simulink model "bh_2dof_ODE_model"  (R2017a)
settings: Solver=ode45  StartTime=0.0  StopTime=20  RelTol=1e-5  EnableMultiTasking=on
PreLoadFcn:
  | bh_script_2dof_params
values from neighbouring files (symbols this model uses):
  c1 = 20    [bh_2dof_MATLAB_analysis.m]
  c2 = 50    [bh_2dof_MATLAB_analysis.m]
  c3 = 10    [bh_2dof_MATLAB_analysis.m]
  k1 = 1000    [bh_2dof_MATLAB_analysis.m]
  k2 = 500    [bh_2dof_MATLAB_analysis.m]
  k3 = 100    [bh_2dof_MATLAB_analysis.m]
  m1 = 10    [bh_2dof_MATLAB_analysis.m]
  m2 = 1    [bh_2dof_MATLAB_analysis.m]
undefined symbols (not defined in the file or in its folder): Cm_mat, init_pos_col, init_vel_col, init_x1, init_x1dot, init_x2, init_x2dot, Km_mat, Mm_mat
settings Model: Creator=bhorton  LastModifiedBy=bhorton
settings OptimizationCC: LifeSpan=inf
settings DebuggingCC: SFUnexpectedBacktrackingDiag=warning  SFNoUnconditionalDefaultTransitionDiag=warning  SFExecutionAtInitializationDiag=none
settings GRTTargetCC: TargetLangStandard=C89/C90 (ANSI)  GeneratePreprocessorConditionals=Disable all
settings ConfigComp: CovMetricSettings=dw  CovHtmlReporting=on  CovSaveCumulativeToWorkspaceVar=on  CovSaveSingleToWorkspaceVar=on  CovExternalEMLEnable=off

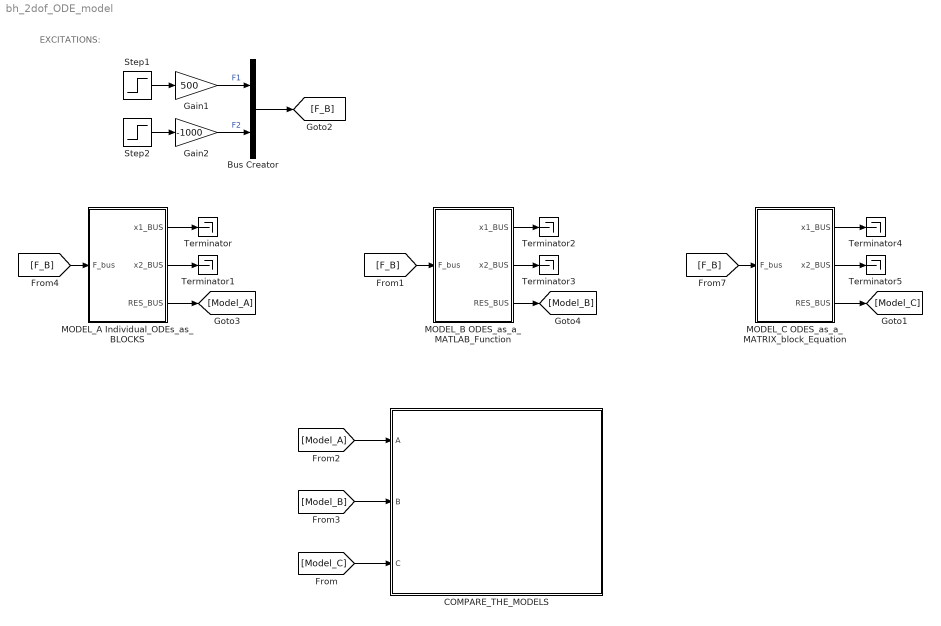
== system bh_2dof_ODE_model ==
  note: EXCITATIONS:
  Bus Creator : BusCreator  Inputs=2
  COMPARE_THE_MODELS : Subsystem
  Gain1 : Gain  Gain=500
  Gain2 : Gain  Gain=-1000
  MODEL_A Individual_ODEs_as_BLOCKS : Subsystem
  "MODEL_B ODES_as_a_MATLAB_Function " : Subsystem
  MODEL_C ODES_as_a_MATRIX_block_Equation : Subsystem
  Step1 : Step  Time=5  SampleTime=0
      settings: AttributesFormatString=Step @ T=%<Time>
  Step2 : Step  Time=10  SampleTime=0
      settings: AttributesFormatString=Step @ T=%<Time>
  Terminator{,1..5} (6 alike) : Terminator
  wires:
  Step1/1 -> Gain1/1
  Gain1/1 -> Bus Creator/1  "F1"
  Step2/1 -> Gain2/1
  Gain2/1 -> Bus Creator/2  "F2"
  Bus Creator/1 -> [F_B]
  [F_B] -> MODEL_A Individual_ODEs_as_BLOCKS/1(F_bus)
  [F_B] -> "MODEL_B ODES_as_a_MATLAB_Function "/1(F_bus)
  [F_B] -> MODEL_C ODES_as_a_MATRIX_block_Equation/1(F_bus)
  MODEL_A Individual_ODEs_as_BLOCKS/3(RES_BUS) -> [Model_A]
  "MODEL_B ODES_as_a_MATLAB_Function "/3(RES_BUS) -> [Model_B]
  MODEL_C ODES_as_a_MATRIX_block_Equation/3(RES_BUS) -> [Model_C]
  [Model_A] -> COMPARE_THE_MODELS/1(A)
  [Model_B] -> COMPARE_THE_MODELS/2(B)
  [Model_C] -> COMPARE_THE_MODELS/3(C)
  MODEL_A Individual_ODEs_as_BLOCKS/1(x1_BUS) -> Terminator/1
  MODEL_A Individual_ODEs_as_BLOCKS/2(x2_BUS) -> Terminator1/1
  "MODEL_B ODES_as_a_MATLAB_Function "/1(x1_BUS) -> Terminator2/1
  "MODEL_B ODES_as_a_MATLAB_Function "/2(x2_BUS) -> Terminator3/1
  MODEL_C ODES_as_a_MATRIX_block_Equation/2(x2_BUS) -> Terminator5/1
  MODEL_C ODES_as_a_MATRIX_block_Equation/1(x1_BUS) -> Terminator4/1

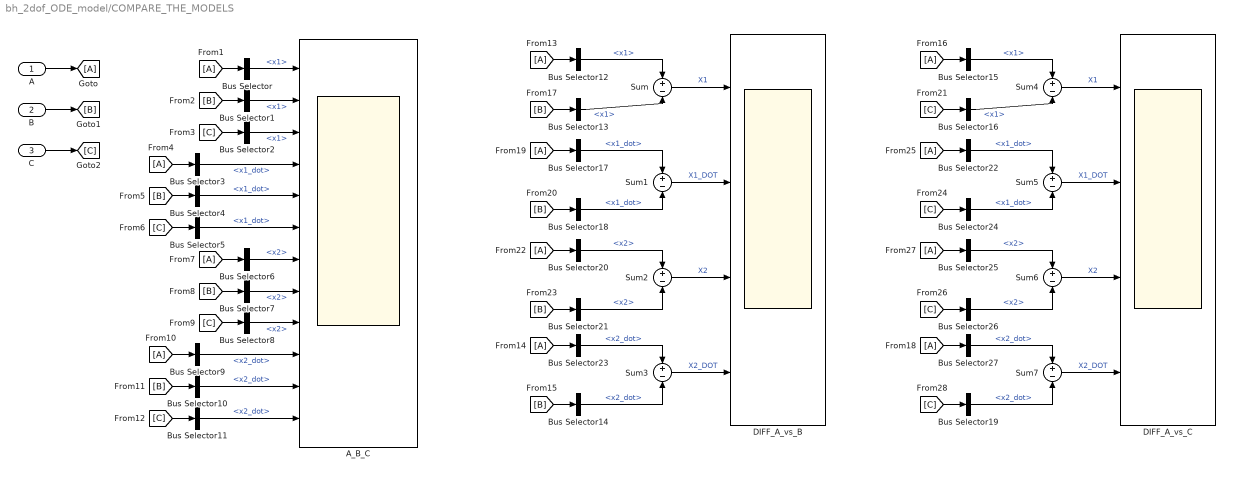
== system bh_2dof_ODE_model/COMPARE_THE_MODELS ==
  A : Inport
  B : Inport  Port=2
  C : Inport  Port=3
  A_B_C : Scope  NumInputPorts=12
  Bus Selector{,1..2,12..13,15..16} (7 alike) : BusSelector  OutputSignals=x1_BUS.x1
  Bus Selector{9..11,14,19,23,27} (7 alike) : BusSelector  OutputSignals=x2_BUS.x2_dot
  Bus Selector{3..5,17..18,22,24} (7 alike) : BusSelector  OutputSignals=x1_BUS.x1_dot
  Bus Selector{6..8,20..21,25..26} (7 alike) : BusSelector  OutputSignals=x2_BUS.x2
  DIFF_A_vs_B : Scope  NumInputPorts=4
  DIFF_A_vs_C : Scope  NumInputPorts=4
  Sum{,1..7} (8 alike) : Sum  Inputs=+|-
  wires:
  A/1 -> [A]
  B/1 -> [B]
  C/1 -> [C]
  [A] -> Bus Selector/1
  [B] -> Bus Selector1/1
  [C] -> Bus Selector2/1
  Bus Selector2/1 -> A_B_C/3  "<x1>"
  Bus Selector1/1 -> A_B_C/2  "<x1>"
  Bus Selector/1 -> A_B_C/1  "<x1>"
  Bus Selector3/1 -> A_B_C/4  "<x1_dot>"
  [A] -> Bus Selector3/1
  [C] -> Bus Selector5/1
  [B] -> Bus Selector4/1
  Bus Selector4/1 -> A_B_C/5  "<x1_dot>"
  Bus Selector5/1 -> A_B_C/6  "<x1_dot>"
  [B] -> Bus Selector7/1
  Bus Selector6/1 -> A_B_C/7  "<x2>"
  [C] -> Bus Selector8/1
  [A] -> Bus Selector6/1
  Bus Selector7/1 -> A_B_C/8  "<x2>"
  Bus Selector8/1 -> A_B_C/9  "<x2>"
  Bus Selector9/1 -> A_B_C/10  "<x2_dot>"
  [A] -> Bus Selector9/1
  [C] -> Bus Selector11/1
  [B] -> Bus Selector10/1
  Bus Selector10/1 -> A_B_C/11  "<x2_dot>"
  Bus Selector11/1 -> A_B_C/12  "<x2_dot>"
  Sum3/1 -> DIFF_A_vs_B/4  "X2_DOT"
  Bus Selector12/1 -> Sum/1  "<x1>"
  [A] -> Bus Selector20/1
  [A] -> Bus Selector17/1
  Bus Selector13/1 -> Sum/2  "<x1>"
  [B] -> Bus Selector14/1
  Bus Selector20/1 -> Sum2/1  "<x2>"
  [A] -> Bus Selector23/1
  [B] -> Bus Selector18/1
  [B] -> Bus Selector13/1
  [B] -> Bus Selector21/1
  Bus Selector14/1 -> Sum3/2  "<x2_dot>"
  Bus Selector18/1 -> Sum1/2  "<x1_dot>"
  Sum2/1 -> DIFF_A_vs_B/3  "X2"
  Bus Selector23/1 -> Sum3/1  "<x2_dot>"
  Sum/1 -> DIFF_A_vs_B/1  "X1"
  Sum1/1 -> DIFF_A_vs_B/2  "X1_DOT"
  Bus Selector17/1 -> Sum1/1  "<x1_dot>"
  Bus Selector21/1 -> Sum2/2  "<x2>"
  [A] -> Bus Selector12/1
  Bus Selector26/1 -> Sum6/2  "<x2>"
  Bus Selector15/1 -> Sum4/1  "<x1>"
  [A] -> Bus Selector15/1
  [C] -> Bus Selector19/1
  [C] -> Bus Selector26/1
  [C] -> Bus Selector16/1
  Sum4/1 -> DIFF_A_vs_C/1  "X1"
  Bus Selector19/1 -> Sum7/2  "<x2_dot>"
  [A] -> Bus Selector22/1
  Sum6/1 -> DIFF_A_vs_C/3  "X2"
  Bus Selector16/1 -> Sum4/2  "<x1>"
  Bus Selector25/1 -> Sum6/1  "<x2>"
  [A] -> Bus Selector27/1
  Bus Selector24/1 -> Sum5/2  "<x1_dot>"
  [A] -> Bus Selector25/1
  [C] -> Bus Selector24/1
  Bus Selector27/1 -> Sum7/1  "<x2_dot>"
  Bus Selector22/1 -> Sum5/1  "<x1_dot>"
  Sum5/1 -> DIFF_A_vs_C/2  "X1_DOT"
  Sum7/1 -> DIFF_A_vs_C/4  "X2_DOT"

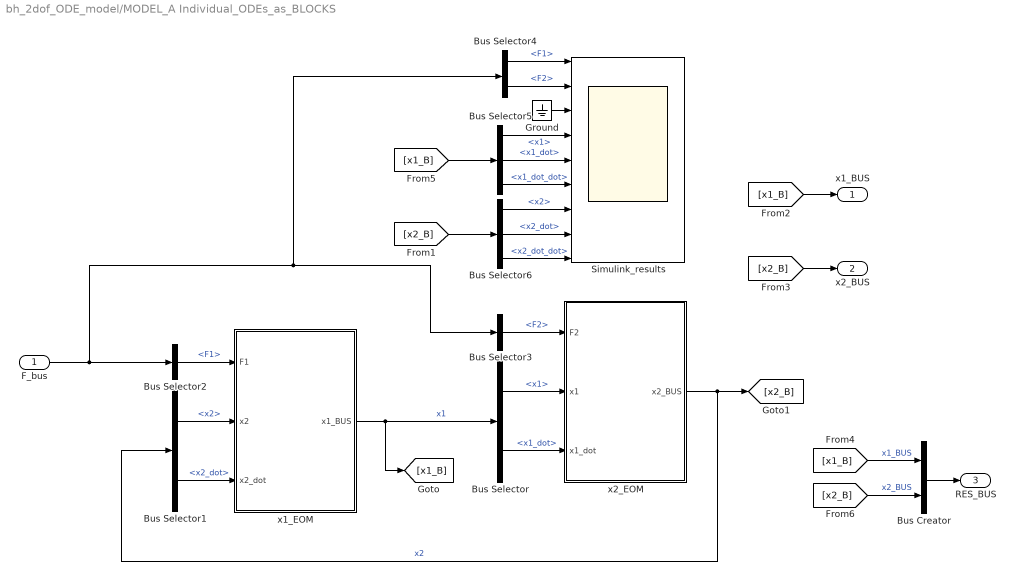
== system bh_2dof_ODE_model/MODEL_A Individual_ODEs_as_BLOCKS ==
  F_bus : Inport
  Bus Creator : BusCreator  Inputs=2
  Bus Selector : BusSelector  OutputSignals=x1,x1_dot
  Bus Selector1 : BusSelector  OutputSignals=x2,x2_dot
  Bus Selector2 : BusSelector  OutputSignals=F1
  Bus Selector3 : BusSelector  OutputSignals=F2
  Bus Selector4 : BusSelector  OutputSignals=F1,F2
  Bus Selector5 : BusSelector  OutputSignals=x1,x1_dot,x1_dot_dot
  Bus Selector6 : BusSelector  OutputSignals=x2,x2_dot,x2_dot_dot
  Ground : Ground
  Simulink_results : Scope  NumInputPorts=9
  x1_EOM : Subsystem
  x2_EOM : Subsystem
  x1_BUS : Outport
  x2_BUS : Outport  Port=2
  RES_BUS : Outport  Port=3
  wires:
  Bus Selector/2 -> x2_EOM/3(x1_dot)  "<x1_dot>"
  Bus Selector/1 -> x2_EOM/2(x1)  "<x1>"
  Bus Selector1/1 -> x1_EOM/2(x2)  "<x2>"
  Bus Selector1/2 -> x1_EOM/3(x2_dot)  "<x2_dot>"
  x1_EOM/1(x1_BUS) -> [x1_B], Bus Selector/1  "x1"
  x2_EOM/1(x2_BUS) -> Bus Selector1/1, [x2_B]  "x2"
  Bus Selector2/1 -> x1_EOM/1(F1)  "<F1>"
  Bus Selector3/1 -> x2_EOM/1(F2)  "<F2>"
  F_bus/1 -> Bus Selector4/1, Bus Selector3/1, Bus Selector2/1
  Bus Selector4/1 -> Simulink_results/1  "<F1>"
  Bus Selector4/2 -> Simulink_results/2  "<F2>"
  Ground/1 -> Simulink_results/3
  [x1_B] -> Bus Selector5/1
  Bus Selector5/3 -> Simulink_results/6  "<x1_dot_dot>"
  Bus Selector5/2 -> Simulink_results/5  "<x1_dot>"
  Bus Selector5/1 -> Simulink_results/4  "<x1>"
  Bus Selector6/1 -> Simulink_results/7  "<x2>"
  Bus Selector6/2 -> Simulink_results/8  "<x2_dot>"
  Bus Selector6/3 -> Simulink_results/9  "<x2_dot_dot>"
  [x2_B] -> Bus Selector6/1
  [x1_B] -> x1_BUS/1
  [x2_B] -> x2_BUS/1
  Bus Creator/1 -> RES_BUS/1
  [x1_B] -> Bus Creator/1  "x1_BUS"
  [x2_B] -> Bus Creator/2  "x2_BUS"

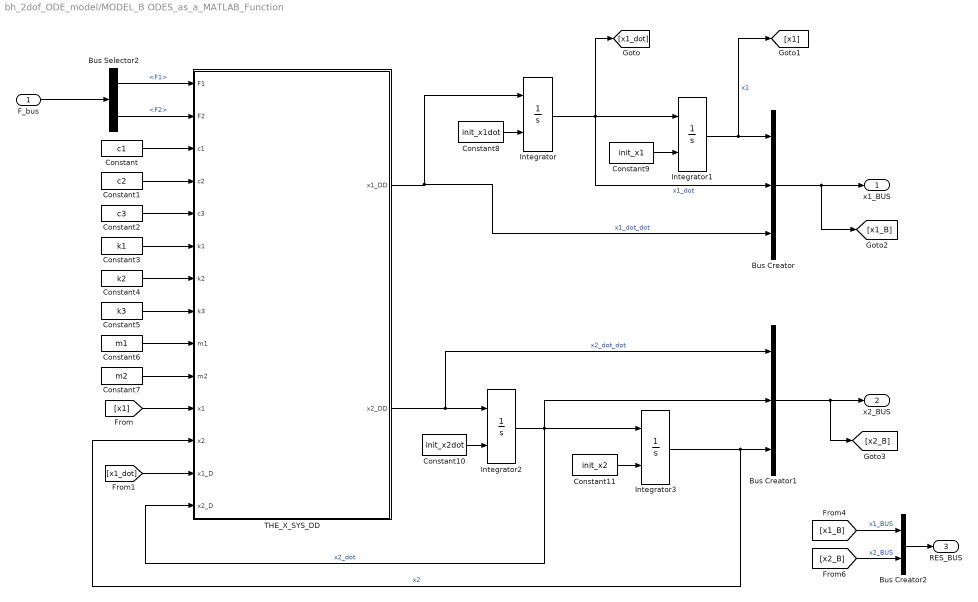
== system bh_2dof_ODE_model/MODEL_B ODES_as_a_MATLAB_Function  ==
  F_bus : Inport
  Bus Creator : BusCreator  Inputs=3
  Bus Creator1 : BusCreator  Inputs=3
  Bus Creator2 : BusCreator  Inputs=2
  Bus Selector2 : BusSelector  OutputSignals=F1,F2
  Constant : Constant  Value=c1
  Constant1 : Constant  Value=c2
  Constant10 : Constant  Value=init_x2dot
  Constant11 : Constant  Value=init_x2
  Constant2 : Constant  Value=c3
  Constant3 : Constant  Value=k1
  Constant4 : Constant  Value=k2
  Constant5 : Constant  Value=k3
  Constant6 : Constant  Value=m1
  Constant7 : Constant  Value=m2
  Constant8 : Constant  Value=init_x1dot
  Constant9 : Constant  Value=init_x1
  Integrator{,1..3} (4 alike) : Integrator  InitialConditionSource=external
  THE_X_SYS_DD : MATLAB Function  TreatAsAtomicUnit=on
  x1_BUS : Outport
  x2_BUS : Outport  Port=2
  RES_BUS : Outport  Port=3
  wires:
  F_bus/1 -> Bus Selector2/1
  Bus Selector2/2 -> THE_X_SYS_DD/2(F2)  "<F2>"
  Bus Selector2/1 -> THE_X_SYS_DD/1(F1)  "<F1>"
  Constant7/1 -> THE_X_SYS_DD/10(m2)
  Constant6/1 -> THE_X_SYS_DD/9(m1)
  Constant5/1 -> THE_X_SYS_DD/8(k3)
  Constant4/1 -> THE_X_SYS_DD/7(k2)
  Constant3/1 -> THE_X_SYS_DD/6(k1)
  Constant2/1 -> THE_X_SYS_DD/5(c3)
  Constant1/1 -> THE_X_SYS_DD/4(c2)
  Constant/1 -> THE_X_SYS_DD/3(c1)
  Bus Creator/1 -> [x1_B], x1_BUS/1
  THE_X_SYS_DD/1(x1_DD) -> Bus Creator/3, Integrator/1  "x1_dot_dot"
  Constant9/1 -> Integrator1/2
  Constant8/1 -> Integrator/2
  Integrator/1 -> [x1_dot], Bus Creator/2, Integrator1/1  "x1_dot"
  Constant11/1 -> Integrator3/2
  THE_X_SYS_DD/2(x2_DD) -> Bus Creator1/1, Integrator2/1  "x2_dot_dot"
  Bus Creator1/1 -> [x2_B], x2_BUS/1
  Integrator3/1 -> Bus Creator1/3, THE_X_SYS_DD/12(x2)  "x2"
  Constant10/1 -> Integrator2/2
  Integrator2/1 -> Bus Creator1/2, Integrator3/1, THE_X_SYS_DD/14(x2_D)  "x2_dot"
  Integrator1/1 -> [x1], Bus Creator/1  "x1"
  [x1] -> THE_X_SYS_DD/11(x1)
  [x1_dot] -> THE_X_SYS_DD/13(x1_D)
  [x1_B] -> Bus Creator2/1  "x1_BUS"
  [x2_B] -> Bus Creator2/2  "x2_BUS"
  Bus Creator2/1 -> RES_BUS/1

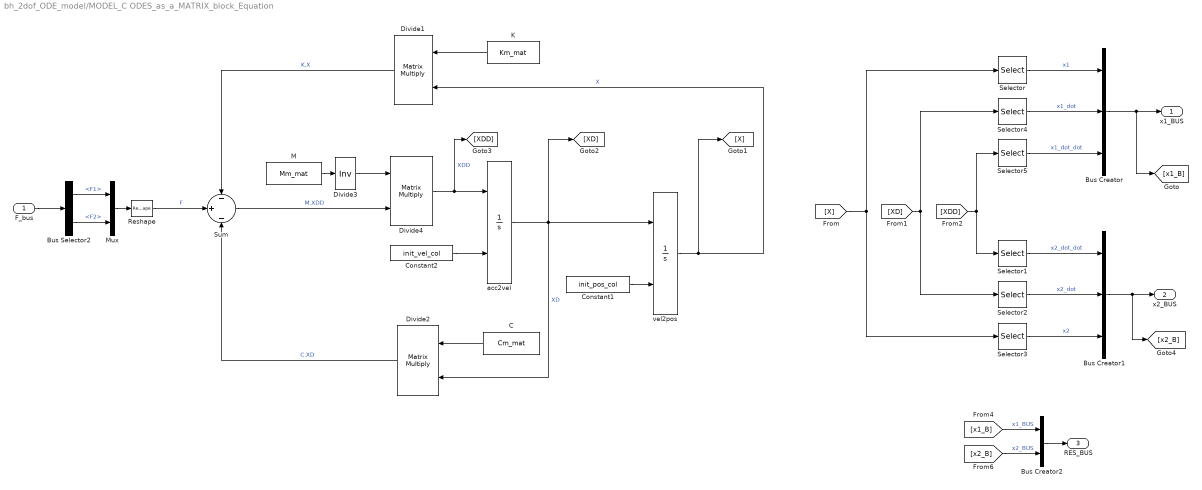
== system bh_2dof_ODE_model/MODEL_C ODES_as_a_MATRIX_block_Equation ==
  F_bus : Inport
  Bus Creator : BusCreator  Inputs=3
  Bus Creator1 : BusCreator  Inputs=3
  Bus Creator2 : BusCreator  Inputs=2
  Bus Selector2 : BusSelector  OutputSignals=F1,F2
  C : Constant  Value=Cm_mat
  Constant1 : Constant  Value=init_pos_col
  Constant2 : Constant  Value=init_vel_col
  Divide1 : Product  Multiplication=Matrix(*)
  Divide2 : Product  Multiplication=Matrix(*)
  Divide3 : Product  Inputs=/  Multiplication=Matrix(*)
  Divide4 : Product  Multiplication=Matrix(*)
  K : Constant  Value=Km_mat
  M : Constant  Value=Mm_mat
  Mux : Mux  Inputs=2
  Reshape : Reshape  OutputDimensionality=Column vector (2-D)
  Selector : Selector  InputPortWidth=2  IndexOptions=Index vector (dialog)  Indices=[1 ]  OutputSizes=1
  Selector1 : Selector  InputPortWidth=2  IndexOptions=Index vector (dialog)  Indices=[2]  OutputSizes=1
  Selector2 : Selector  InputPortWidth=2  IndexOptions=Index vector (dialog)  Indices=[2]  OutputSizes=1
  Selector3 : Selector  InputPortWidth=2  IndexOptions=Index vector (dialog)  Indices=[2]  OutputSizes=1
  Selector4 : Selector  InputPortWidth=2  IndexOptions=Index vector (dialog)  Indices=[1 ]  OutputSizes=1
  Selector5 : Selector  InputPortWidth=2  IndexOptions=Index vector (dialog)  Indices=[1 ]  OutputSizes=1
  Sum : Sum  Inputs=-|+|-
  acc2vel : Integrator  InitialConditionSource=external
  vel2pos : Integrator  InitialConditionSource=external
  x1_BUS : Outport
  x2_BUS : Outport  Port=2
  RES_BUS : Outport  Port=3
  wires:
  F_bus/1 -> Bus Selector2/1
  Bus Selector2/2 -> Mux/2  "<F2>"
  Bus Selector2/1 -> Mux/1  "<F1>"
  Bus Creator/1 -> [x1_B], x1_BUS/1
  Bus Creator1/1 -> [x2_B], x2_BUS/1
  Mux/1 -> Reshape/1
  Reshape/1 -> Sum/2  "F"
  K/1 -> Divide1/1
  C/1 -> Divide2/1
  Divide2/1 -> Sum/3  "C.XD"
  Divide1/1 -> Sum/1  "K.X"
  Sum/1 -> Divide4/2  "M.XDD"
  M/1 -> Divide3/1
  Divide3/1 -> Divide4/1
  Divide4/1 -> [XDD], acc2vel/1  "XDD"
  Constant2/1 -> acc2vel/2
  acc2vel/1 -> [XD], vel2pos/1, Divide2/2  "XD"
  Constant1/1 -> vel2pos/2
  vel2pos/1 -> [X], Divide1/2  "X"
  Selector5/1 -> Bus Creator/3  "x1_dot_dot"
  Selector4/1 -> Bus Creator/2  "x1_dot"
  Selector/1 -> Bus Creator/1  "x1"
  [XDD] -> Selector5/1, Selector1/1
  [XD] -> Selector2/1, Selector4/1
  [X] -> Selector/1, Selector3/1
  Selector1/1 -> Bus Creator1/1  "x2_dot_dot"
  Selector2/1 -> Bus Creator1/2  "x2_dot"
  Selector3/1 -> Bus Creator1/3  "x2"
  Bus Creator2/1 -> RES_BUS/1
  [x1_B] -> Bus Creator2/1  "x1_BUS"
  [x2_B] -> Bus Creator2/2  "x2_BUS"

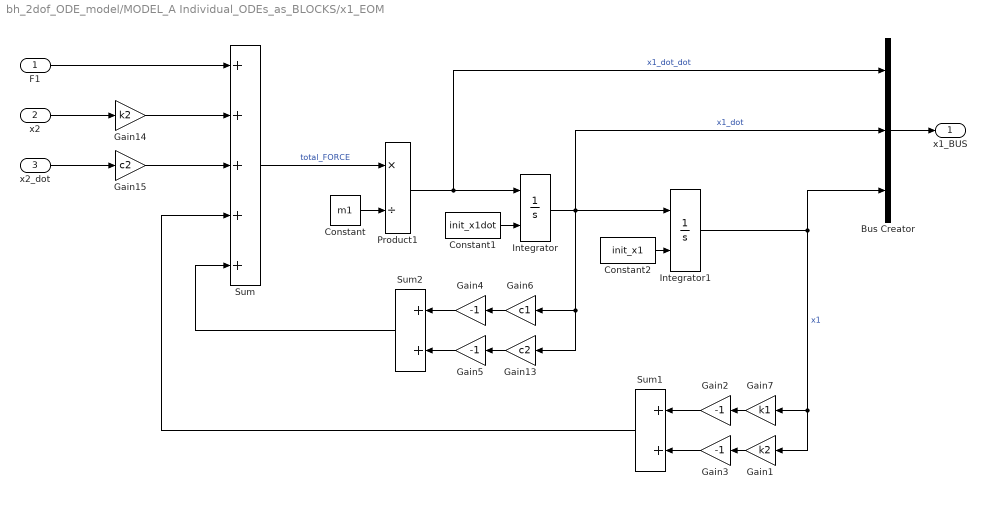
== system bh_2dof_ODE_model/MODEL_A Individual_ODEs_as_BLOCKS/x1_EOM ==
  F1 : Inport
  x2 : Inport  Port=2
  x2_dot : Inport  Port=3
  Bus Creator : BusCreator  Inputs=3
  Constant : Constant  Value=m1
  Constant1 : Constant  Value=init_x1dot
  Constant2 : Constant  Value=init_x1
  Gain1 : Gain  Gain=k2
  Gain13 : Gain  Gain=c2
  Gain14 : Gain  Gain=k2
  Gain15 : Gain  Gain=c2
  Gain{2..5} (4 alike) : Gain  Gain=-1
  Gain6 : Gain  Gain=c1
  Gain7 : Gain  Gain=k1
  Integrator : Integrator  InitialConditionSource=external
  Integrator1 : Integrator  InitialConditionSource=external
  Product1 : Product  Inputs=*/
  Sum : Sum  Inputs=+|+|+|+|+
  Sum1 : Sum  Inputs=2
  Sum2 : Sum  Inputs=2
  x1_BUS : Outport
  wires:
  F1/1 -> Sum/1
  Gain3/1 -> Sum1/2
  Gain4/1 -> Sum2/1
  Gain14/1 -> Sum/2
  Gain6/1 -> Gain4/1
  x2/1 -> Gain14/1
  Gain2/1 -> Sum1/1
  Sum2/1 -> Sum/5
  Sum1/1 -> Sum/4
  x2_dot/1 -> Gain15/1
  Gain15/1 -> Sum/3
  Constant/1 -> Product1/2
  Sum/1 -> Product1/1  "total_FORCE"
  Integrator/1 -> Bus Creator/2, Integrator1/1, Gain13/1, Gain6/1  "x1_dot"
  Product1/1 -> Bus Creator/1, Integrator/1  "x1_dot_dot"
  Integrator1/1 -> Bus Creator/3, Gain7/1, Gain1/1  "x1"
  Bus Creator/1 -> x1_BUS/1
  Gain7/1 -> Gain2/1
  Gain1/1 -> Gain3/1
  Gain5/1 -> Sum2/2
  Gain13/1 -> Gain5/1
  Constant1/1 -> Integrator/2
  Constant2/1 -> Integrator1/2

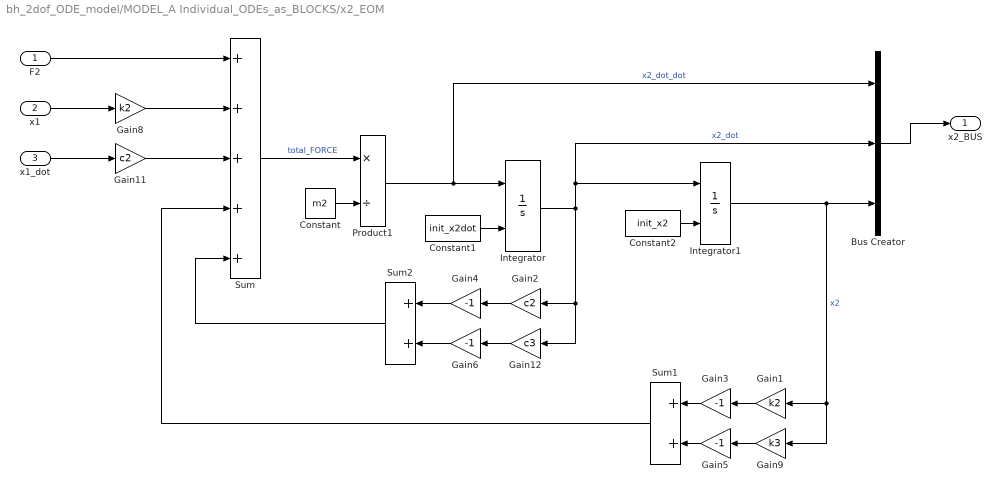
== system bh_2dof_ODE_model/MODEL_A Individual_ODEs_as_BLOCKS/x2_EOM ==
  F2 : Inport
  x1 : Inport  Port=2
  x1_dot : Inport  Port=3
  Bus Creator : BusCreator  Inputs=3
  Constant : Constant  Value=m2
  Constant1 : Constant  Value=init_x2dot
  Constant2 : Constant  Value=init_x2
  Gain1 : Gain  Gain=k2
  Gain11 : Gain  Gain=c2
  Gain12 : Gain  Gain=c3
  Gain2 : Gain  Gain=c2
  Gain{3..6} (4 alike) : Gain  Gain=-1
  Gain8 : Gain  Gain=k2
  Gain9 : Gain  Gain=k3
  Integrator : Integrator  InitialConditionSource=external
  Integrator1 : Integrator  InitialConditionSource=external
  Product1 : Product  Inputs=*/
  Sum : Sum  Inputs=+|+|+|+|+
  Sum1 : Sum  Inputs=2
  Sum2 : Sum  Inputs=2
  x2_BUS : Outport
  wires:
  F2/1 -> Sum/1
  Gain9/1 -> Gain5/1
  Gain4/1 -> Sum2/1
  Gain8/1 -> Sum/2
  x1/1 -> Gain8/1
  Gain12/1 -> Gain6/1
  Sum2/1 -> Sum/5
  Sum1/1 -> Sum/4
  x1_dot/1 -> Gain11/1
  Gain11/1 -> Sum/3
  Constant/1 -> Product1/2
  Sum/1 -> Product1/1  "total_FORCE"
  Integrator/1 -> Integrator1/1, Bus Creator/2, Gain12/1, Gain2/1  "x2_dot"
  Product1/1 -> Bus Creator/1, Integrator/1  "x2_dot_dot"
  Integrator1/1 -> Bus Creator/3, Gain9/1, Gain1/1  "x2"
  Gain3/1 -> Sum1/1
  Gain1/1 -> Gain3/1
  Gain2/1 -> Gain4/1
  Bus Creator/1 -> x2_BUS/1
  Gain5/1 -> Sum1/2
  Gain6/1 -> Sum2/2
  Constant1/1 -> Integrator/2
  Constant2/1 -> Integrator1/2

== matlab function bh_2dof_ODE_model/MODEL_B ODES_as_a_MATLAB_Function /THE_X_SYS_DD ==
  data: F1 input; x1_DD output; F2 input; c1 input; c2 input; c3 input; k1 input; k2 input; k3 input; m1 input; m2 input; x1 input; x2 input; x1_D input; x2_D input; x2_DD output
function [x1_DD,x2_DD] = THE_X_SYS_DD(F1,F2,c1,c2,c3,k1,k2,k3,m1,m2,x1,x2,x1_D,x2_D)
%#codegen

%    This function was generated by the Symbolic Math Toolbox version 7.2.
%    03-Apr-2017 09:10:59

x1_DD = -(-F1+c1.*x1_D+c2.*x1_D-c2.*x2_D+k1.*x1+k2.*x1-k2.*x2)./m1;
if nargout > 1
    x2_DD = -(-F2-c2.*x1_D+c2.*x2_D+c3.*x2_D-k2.*x1+k2.*x2+k3.*x2)./m2;
end
